simulink model "fuzzy_r"  (R2015b)
settings: Solver=VariableStepAuto  StartTime=0.0  StopTime=10.0  RelTol=1e-3
libraries: fuzblock x1, simulink x1
settings Model: Creator=Hp  LastModifiedBy=Hp
settings DataIOCC: LimitDataPoints=off
settings DebuggingCC: AllowSymbolicDim=on
settings ModelReferenceCC: PropagateSignalLabelsOutOfModel=on
settings GRTTargetCC: GeneratePreprocessorConditionals=Disable all

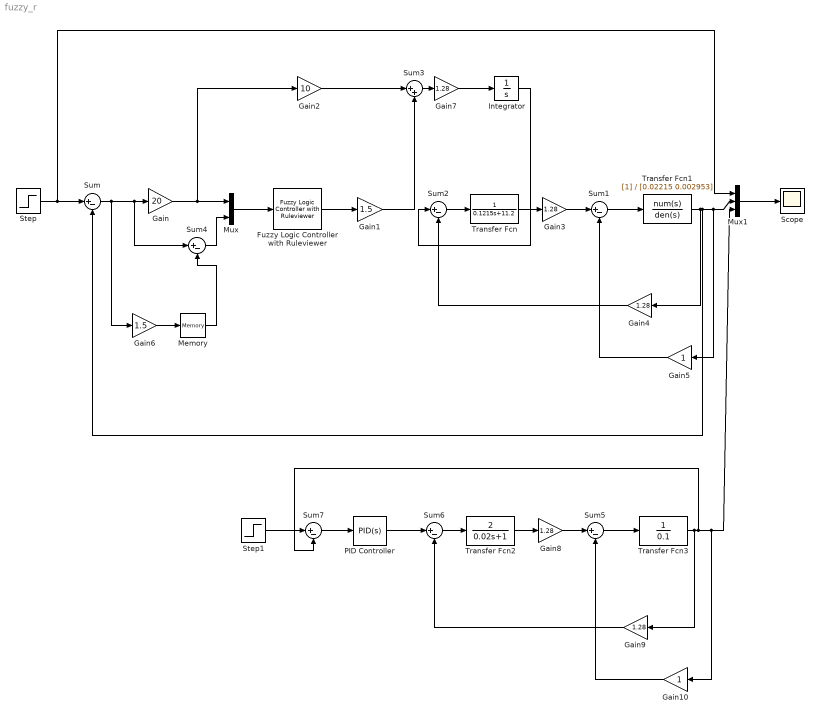
== system fuzzy_r ==
  Fuzzy Logic Controller with Ruleviewer : fuzblock/Fuzzy Logic  Controller  with Ruleviewer  fismatrix=motor_control  Ts=2
  Gain : Gain  Gain=20
  Gain1 : Gain  Gain=1.5
  Gain10 : Gain
  Gain2 : Gain  Gain=10
  Gain{3..4,7..9} (5 alike) : Gain  Gain=1.28
  Gain5 : Gain
  Gain6 : Gain  Gain=1.5
  Integrator : Integrator
  Memory : Memory
  Mux : Mux  Inputs=2
  Mux1 : Mux  Inputs=3
  PID Controller : simulink/Continuous/PID Controller  Controller=PID  TimeDomain=Continuous-time  SampleTime=-1  IntegratorMethod=Forward Euler  FilterMethod=Forward Euler  Form=Parallel  UseFilter=on  ControllerParametersSource=internal  P=2.287  I=909.4  D=-0.000417449068520689  N=752.201155532888  InitialConditionSource=internal  InitialConditionForIntegrator=0  InitialConditionForFilter=0  ExternalReset=none  LimitOutput=off  UpperSaturationLimit=inf  LowerSaturationLimit=-inf  LinearizeAsGain=on  AntiWindupMode=none  Kb=1  TrackingMode=off  Kt=1  PParamMin=[]  PParamMax=[]  IParamMin=[]  IParamMax=[]  DParamMin=[]  DParamMax=[]  NParamMin=[]  NParamMax=[]  KbParamMin=[]  KbParamMax=[]  KtParamMin=[]  KtParamMax=[]  POutMin=[]  POutMax=[]  IOutMin=[]  IOutMax=[]  DOutMin=[]  DOutMax=[]  NOutMin=[]  NOutMax=[]  KbOutMin=[]  KbOutMax=[]  KtOutMin=[]  KtOutMax=[]  IntegratorOutMin=[]  IntegratorOutMax=[]  FilterOutMin=[]  FilterOutMax=[]  SumOutMin=[]  SumOutMax=[]  SumI1OutMin=[]  SumI1OutMax=[]  SumI2OutMin=[]  SumI2OutMax=[]  SumI3OutMin=[]  SumI3OutMax=[]  SumDOutMin=[]  SumDOutMax=[]  SaturationOutMin=[]  SaturationOutMax=[]  IntegratorContinuousStateAttributes=''  IntegratorStateMustResolveToSignalObject=off  IntegratorRTWStateStorageClass=Auto  FilterContinuousStateAttributes=''  FilterStateMustResolveToSignalObject=off  FilterRTWStateStorageClass=Auto  DifferentiatorICPrevScaledInput=0  DifferentiatorOutMin=[]  DifferentiatorOutMax=[]
  Scope : Scope
  Step : Step  Time=0.5  SampleTime=0
  Step1 : Step  Time=0.5  SampleTime=0
  Sum{,1..2,4..7} (7 alike) : Sum  Inputs=|+-
  Sum3 : Sum  Inputs=|++
  Transfer Fcn : TransferFcn  Denominator=[0.1215 11.2]
  Transfer Fcn1 : TransferFcn  Denominator=[0.02215 0.002953]
  Transfer Fcn2 : TransferFcn  Numerator=[2]  Denominator=[0.02 1]
  Transfer Fcn3 : TransferFcn  Denominator=[0.1]
  wires:
  Gain3/1 -> Sum1/1
  Sum1/1 -> Transfer Fcn1/1
  Step/1 -> Mux1/1, Sum/1
  Sum/1 -> Gain6/1, Sum4/1, Gain/1
  Sum4/1 -> Mux/2
  Gain/1 -> Gain2/1, Mux/1
  Mux/1 -> Fuzzy Logic Controller with Ruleviewer/1
  Fuzzy Logic Controller with Ruleviewer/1 -> Gain1/1
  Gain1/1 -> Sum3/2
  Gain2/1 -> Sum3/1
  Integrator/1 -> Sum2/1
  Gain4/1 -> Sum2/2
  Sum2/1 -> Transfer Fcn/1
  Transfer Fcn/1 -> Gain3/1
  Transfer Fcn1/1 -> Gain4/1, Gain5/1, Mux1/2, Sum/2
  Gain5/1 -> Sum1/2
  Mux1/1 -> Scope/1
  Sum3/1 -> Gain7/1
  Gain7/1 -> Integrator/1
  Gain6/1 -> Memory/1
  Memory/1 -> Sum4/2
  Gain8/1 -> Sum5/1
  Sum5/1 -> Transfer Fcn3/1
  Gain9/1 -> Sum6/2
  Sum6/1 -> Transfer Fcn2/1
  Transfer Fcn2/1 -> Gain8/1
  Gain10/1 -> Sum5/2
  Transfer Fcn3/1 -> Gain9/1, Gain10/1, Mux1/3, Sum7/2
  Step1/1 -> Sum7/1
  Sum7/1 -> PID Controller/1
  PID Controller/1 -> Sum6/1
